simulink model "pendulodoble"  (R2024a)
settings: Solver=VariableStepAuto  StartTime=0.0  StopTime=10.0  RelTol=1e-3

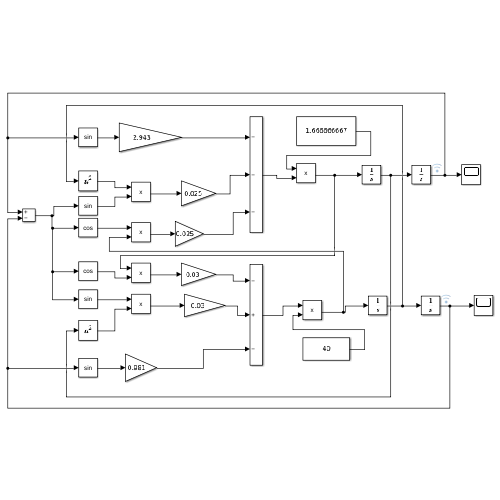
[thumbnail: Simulink's stored preview of the top-level diagram]
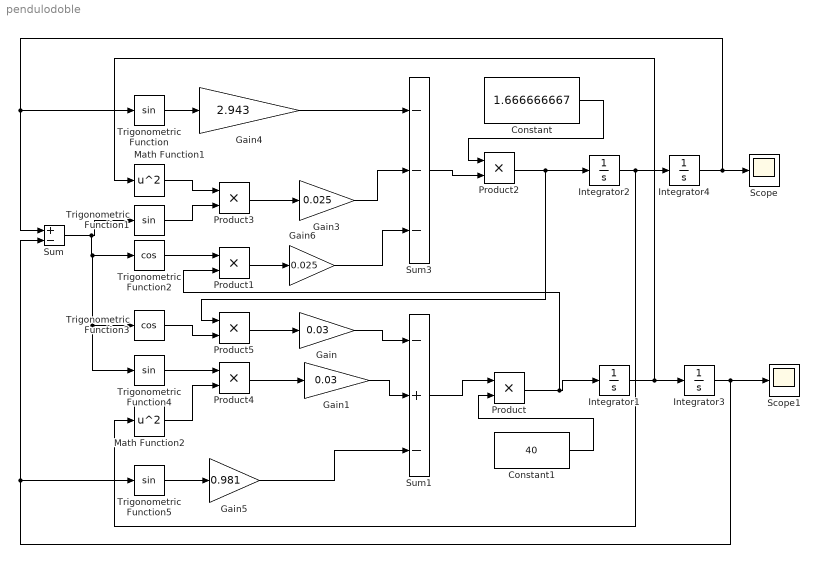
== system pendulodoble ==
  Constant : Constant  Value=1.666666667
  Constant1 : Constant  Value=40
  Gain : Gain  Gain=0.03
  Gain1 : Gain  Gain=0.03
  Gain3 : Gain  Gain=0.025
  Gain4 : Gain  Gain=2.943
  Gain5 : Gain  Gain=0.981
  Gain6 : Gain  Gain=0.025
  Integrator1 : Integrator  InitialCondition=35
  Integrator2 : Integrator
  Integrator3 : Integrator
  Integrator4 : Integrator
  Math Function1 : Math  Operator=square
  Math Function2 : Math  Operator=square
  Product{,1..5} (6 alike) : Product
  Scope : Scope
  Scope1 : Scope
  Sum : Sum  Inputs=+-
  Sum1 : Sum  Inputs=-+-
  Sum3 : Sum  Inputs=---
  Trigonometric Function{,1,4..5} (4 alike) : Trigonometry
  Trigonometric Function2 : Trigonometry  Operator=cos
  Trigonometric Function3 : Trigonometry  Operator=cos
  wires:
  Trigonometric Function/1 -> Gain4/1
  Math Function1/1 -> Product3/1
  Trigonometric Function1/1 -> Product3/2
  Trigonometric Function2/1 -> Product1/1
  Product3/1 -> Gain3/1
  Product1/1 -> Gain6/1
  Gain4/1 -> Sum3/1
  Gain3/1 -> Sum3/2
  Gain6/1 -> Sum3/3
  Sum3/1 -> Product2/2
  Constant/1 -> Product2/1
  Trigonometric Function3/1 -> Product5/2
  Trigonometric Function4/1 -> Product4/1
  Math Function2/1 -> Product4/2
  Trigonometric Function5/1 -> Gain5/1
  Product4/1 -> Gain1/1
  Product5/1 -> Gain/1
  Gain/1 -> Sum1/1
  Gain1/1 -> Sum1/2
  Gain5/1 -> Sum1/3
  Sum1/1 -> Product/1
  Constant1/1 -> Product/2
  Product/1 -> Product1/2, Integrator1/1
  Integrator1/1 -> Math Function1/1, Integrator3/1
  Product2/1 -> Product5/1, Integrator2/1
  Integrator4/1 -> Sum/1, Trigonometric Function/1, Scope/1
  Integrator3/1 -> Trigonometric Function5/1, Sum/2, Scope1/1
  Sum/1 -> Trigonometric Function4/1, Trigonometric Function3/1, Trigonometric Function2/1, Trigonometric Function1/1
  Integrator2/1 -> Math Function2/1, Integrator4/1
